simulink model "FastMPC_Controller"  (R2023b)
settings: Solver=VariableStepAuto  StartTime=0.0  StopTime=20.0  RelTol=1e-3
settings Model: Creator=patel  LastModifiedBy=patel

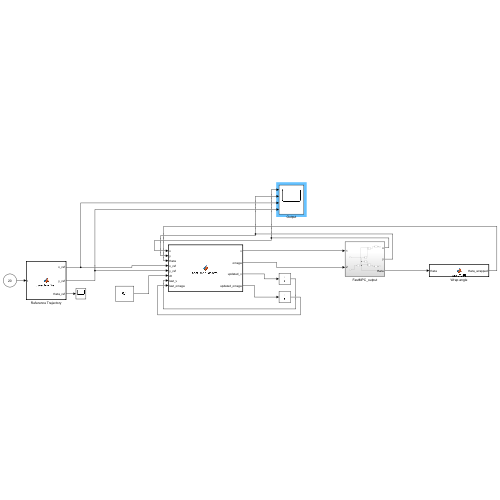
[thumbnail: Simulink's stored preview of the top-level diagram]
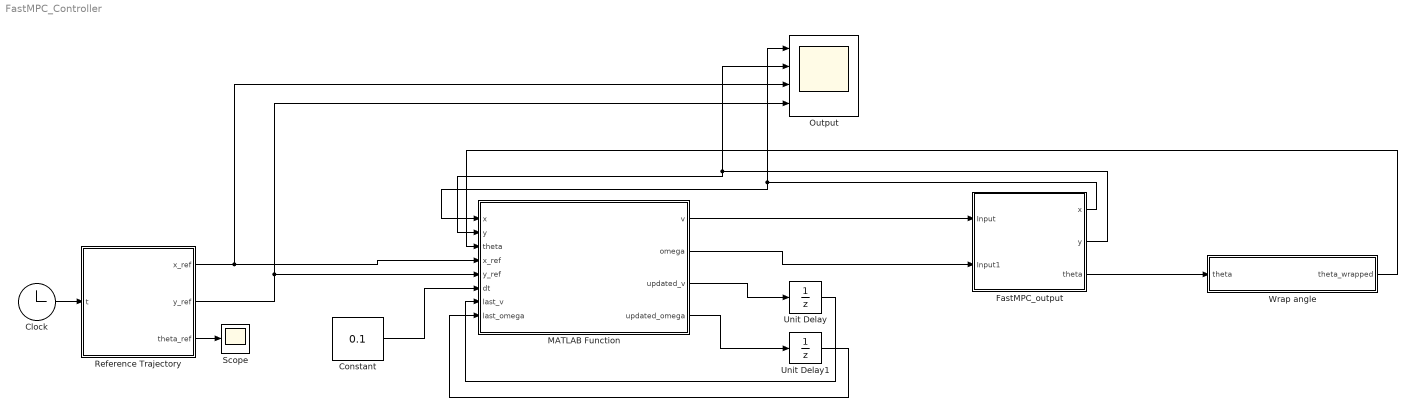
== system FastMPC_Controller ==
  Clock : Clock
      settings: Decimation=20
  Constant : Constant  Value=0.1
  FastMPC_output : Subsystem
  MATLAB Function : MATLAB Function  TreatAsAtomicUnit=on
  Output : Scope  NumInputPorts=4
  Reference Trajectory : MATLAB Function  TreatAsAtomicUnit=on
  Scope : Scope
  Unit Delay : UnitDelay  SampleTime=-1  HasFrameUpgradeWarning=on
  Unit Delay1 : UnitDelay  SampleTime=-1  HasFrameUpgradeWarning=on
  Wrap angle : MATLAB Function  TreatAsAtomicUnit=on
  wires:
  Unit Delay1/1 -> MATLAB Function/8(last_omega)
  Unit Delay/1 -> MATLAB Function/7(last_v)
  Reference Trajectory/2(y_ref) -> Output/4, MATLAB Function/5(y_ref)
  FastMPC_output/1(x) -> MATLAB Function/1(x), Output/1
  FastMPC_output/3(theta) -> Wrap angle/1(theta)
  MATLAB Function/3(updated_v) -> Unit Delay/1
  Reference Trajectory/1(x_ref) -> Output/3, MATLAB Function/4(x_ref)
  Constant/1 -> MATLAB Function/6(dt)
  MATLAB Function/2(omega) -> FastMPC_output/2(Input1)
  MATLAB Function/1(v) -> FastMPC_output/1(Input)
  FastMPC_output/2(y) -> MATLAB Function/2(y), Output/2
  Wrap angle/1(theta_wrapped) -> MATLAB Function/3(theta)
  Reference Trajectory/3(theta_ref) -> Scope/1
  MATLAB Function/4(updated_omega) -> Unit Delay1/1
  Clock/1 -> Reference Trajectory/1(t)

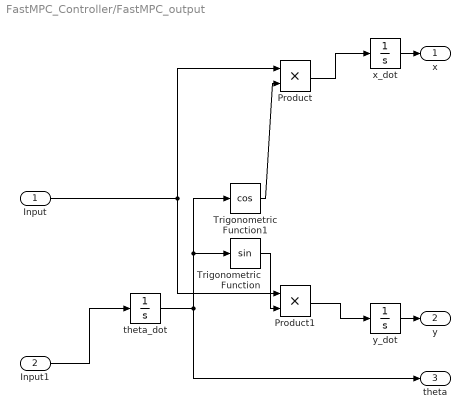
== system FastMPC_Controller/FastMPC_output ==
  Input : Inport
  Input1 : Inport  Port=2
  Product : Product
  Product1 : Product
  Trigonometric Function : Trigonometry
  Trigonometric Function1 : Trigonometry  Operator=cos
  theta_dot : Integrator
  x_dot : Integrator
  y_dot : Integrator
  x : Outport
  y : Outport  Port=2
  theta : Outport  Port=3
  wires:
  theta_dot/1 -> theta/1, Trigonometric Function1/1, Trigonometric Function/1
  Product/1 -> x_dot/1
  Input1/1 -> theta_dot/1
  Trigonometric Function1/1 -> Product/2
  Input/1 -> Product1/1, Product/1
  Trigonometric Function/1 -> Product1/2
  Product1/1 -> y_dot/1
  x_dot/1 -> x/1
  y_dot/1 -> y/1

== matlab function FastMPC_Controller/Reference Trajectory ==
  data: t input; x_ref output; y_ref output; theta_ref output
function [x_ref, y_ref, theta_ref] = trajectoryGen(t)
    radius = 5;
    omega_ref = 0.2;
    x_ref = radius * cos(omega_ref * t);
    y_ref = radius * sin(omega_ref * t);
    theta_ref = omega_ref * t + pi/2;
end

== matlab function FastMPC_Controller/Wrap angle ==
  data: theta input; theta_wrapped output
function theta_wrapped = wrapToPi(theta)
    theta_wrapped = mod(theta + pi, 2*pi) - pi;
end

== matlab function FastMPC_Controller/MATLAB Function ==
  data: x input; v output; y input; theta input; x_ref input; y_ref input; dt input; last_v input; omega output; updated_v output; last_omega input; updated_omega output

function [v, omega, updated_v, updated_omega] = fast_mpc_control(x, y, theta, x_ref, y_ref, dt, last_v, last_omega)
%#codegen
robotState = [x; y; theta];
targetPoint = [x_ref; y_ref];
[v, omega, updated_v, updated_omega] = FastMPCController(robotState, targetPoint, dt, last_v, last_omega);

function [best_v, best_omega, last_v, last_omega] = FastMPCController(robotState, targetPoint, dt, last_v, last_omega)
    % Unpack current state
    x = robotState(1);
    y = robotState(2);
    theta = robotState(3);

    x_target = targetPoint(1);
    y_target = targetPoint(2);

    % MPC parameters
    N = 20;  % Prediction horizon

    % Cost weights (speed-prioritized)
    w_pos = 0.5;
    w_theta = 1.0;
    w_v = 0.05;
    w_omega = 0.1;
    velocity_bias = 0.3;  % Reward for high velocity

    % Control limits
    v_min = 0.0;
    v_max = 5.0;
    omega_min = -pi;
    omega_max = pi;

    % Control search ranges (favoring acceleration)
    v_range_min = max(v_min, last_v - 0.3);
    v_range_max = min(v_max, last_v + 0.7);
    v_options = linspace(v_range_min, v_range_max, 5);
    omega_options = linspace(max(omega_min, last_omega - 0.5), min(omega_max, last_omega + 0.5), 7);

    % Initialize best control
    best_cost = inf;
    best_v = last_v;
    best_omega = last_omega;

    for vi = 1:length(v_options)
        for wi = 1:length(omega_options)
            v = v_options(vi);
            omega = omega_options(wi);

            pred_x = x;
            pred_y = y;
            pred_theta = theta;
            total_cost = 0;

            for i = 0:N-1
                % Predict next state
                pred_x = pred_x + v * cos(pred_theta) * dt;
                pred_y = pred_y + v * sin(pred_theta) * dt;
                pred_theta = pred_theta + omega * dt;

                % Errors
                pos_error = sqrt((x_target - pred_x)^2 + (y_target - pred_y)^2);
                desired_theta = atan2(y_target - pred_y, x_target - pred_x);
                theta_error = atan2(sin(desired_theta - pred_theta), cos(desired_theta - pred_theta));

                % Smoothness
                v_change = abs(v - last_v);
                omega_change = abs(omega - last_omega);

                % Reward for speed
                velocity_reward = -velocity_bias * v / v_max;

                % Step cost
                step_cost = w_pos * pos_error + w_theta * abs(theta_error) + w_v * v_change + w_omega * omega_change + velocity_reward;
                discount = 0.9 ^ i;
                total_cost = total_cost + discount * step_cost;
            end

            % Update best control
            if total_cost < best_cost
                best_cost = total_cost;
                best_v = v;
                best_omega = omega;
            end
        end
    end

    % Update memory for next call
    last_v = best_v;
    last_omega = best_omega;
end
end
